simulink model "AVR_PID"  (R2016a)
settings: Solver=VariableStepAuto  StartTime=0.0  StopTime=10.0  RelTol=1e-3
libraries: simulink x1
settings Model: Creator=EBUKA  LastModifiedBy=EBUKA
settings GRTTargetCC: GeneratePreprocessorConditionals=Use local settings

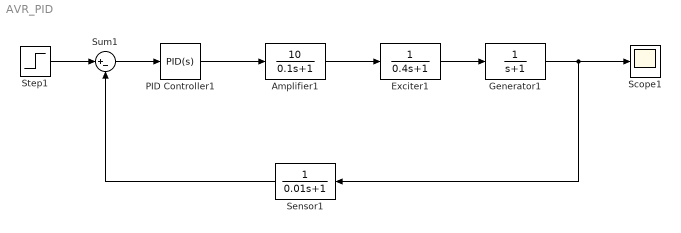
== system AVR_PID ==
  Amplifier1 : TransferFcn  Numerator=[10]  Denominator=[0.1 1]
  Exciter1 : TransferFcn  Denominator=[0.4 1]
  Generator1 : TransferFcn  Denominator=[1 1]
  PID Controller1 : simulink/Continuous/PID Controller  Controller=PID  TimeDomain=Continuous-time  SampleTime=-1  IntegratorMethod=Forward Euler  FilterMethod=Forward Euler  Form=Parallel  UseFilter=on  ControllerParametersSource=internal  P=1.0006  I=0.69306  D=0.31389  N=100  InitialConditionSource=internal  InitialConditionForIntegrator=0  InitialConditionForFilter=0  ExternalReset=none  LimitOutput=off  UpperSaturationLimit=inf  LowerSaturationLimit=-inf  LinearizeAsGain=on  AntiWindupMode=none  Kb=1  TrackingMode=off  Kt=1  PParamMin=[]  PParamMax=[]  IParamMin=[]  IParamMax=[]  DParamMin=[]  DParamMax=[]  NParamMin=[]  NParamMax=[]  KbParamMin=[]  KbParamMax=[]  KtParamMin=[]  KtParamMax=[]  POutMin=[]  POutMax=[]  IOutMin=[]  IOutMax=[]  DOutMin=[]  DOutMax=[]  NOutMin=[]  NOutMax=[]  KbOutMin=[]  KbOutMax=[]  KtOutMin=[]  KtOutMax=[]  IntegratorOutMin=[]  IntegratorOutMax=[]  FilterOutMin=[]  FilterOutMax=[]  SumOutMin=[]  SumOutMax=[]  SumI1OutMin=[]  SumI1OutMax=[]  SumI2OutMin=[]  SumI2OutMax=[]  SumI3OutMin=[]  SumI3OutMax=[]  SumDOutMin=[]  SumDOutMax=[]  SaturationOutMin=[]  SaturationOutMax=[]  IntegratorContinuousStateAttributes=''  IntegratorStateMustResolveToSignalObject=off  IntegratorRTWStateStorageClass=Auto  FilterContinuousStateAttributes=''  FilterStateMustResolveToSignalObject=off  FilterRTWStateStorageClass=Auto  DifferentiatorICPrevScaledInput=0  DifferentiatorOutMin=[]  DifferentiatorOutMax=[]
  Scope1 : Scope
  Sensor1 : TransferFcn  Denominator=[0.01 1]
  Step1 : Step  Time=0  SampleTime=0
  Sum1 : Sum  Inputs=|+-
  wires:
  Exciter1/1 -> Generator1/1
  Amplifier1/1 -> Exciter1/1
  Generator1/1 -> Scope1/1, Sensor1/1
  Sensor1/1 -> Sum1/2
  Step1/1 -> Sum1/1
  PID Controller1/1 -> Amplifier1/1
  Sum1/1 -> PID Controller1/1
